simulink model "staticCalibrationDataGenerator"  (R2023b)
settings: Solver=VariableStepAuto  StartTime=0.0  StopTime=20  RelTol=1e-3
values from neighbouring files (symbols this model uses):
  acc_bias = [2*(rand-0.5)*acc_xy_bias_tolerance 2*(rand-0.5)*acc_xy_bias_tolerance 2*(rand-0.5)*acc_z_bias_tolerance]    [sim_cfg.m]
  acc_bias_over_temp = 2*(rand([1 3])-0.5)*acc_bias_over_temp_tolerance    [sim_cfg.m]
  acc_dynamic = 2*9.81    (= 19.62)    [sim_cfg.m]
  acc_freq = 100    [sim_cfg.m]
  acc_gain_over_temp = diag(2*(rand([1 3])-0.5)*acc_bias_over_temp_tolerance)    [sim_cfg.m]
  acc_noise = 0.008*9.81    (= 0.07848)    [sim_cfg.m]
  acc_non_orthogonality = acc_axis_alignement*acc_non_orthogonality    [sim_cfg.m]
  beac1_pos = [0.1 0 0]    [sim_cfg.m]
  beac2_pos = [-0.1 0 0]    [sim_cfg.m]
  cam1_k = X(39)    [calib2.m]    (also in der.m = C(8); sim_cfg.m = cam_res/(2*tan((cam_AoV+(rand-0.5)*cam_AoV_accur)/2)))
  cam1_orientation_q = angle2quat(cam1_orientation(1),cam1_orientation(2),cam1_orientation(3))    [sim_cfg.m]
  cam1_position = cam1_mounting_position+(rand([1 3])-0.5)*cam_mounting_accur_pos    [sim_cfg.m]
  cam2_k = X(47)    [calib2.m]    (also in der.m = C(16); sim_cfg.m = cam_res/(2*tan((cam_AoV+(rand-0.5)*cam_AoV_accur)/2)))
  cam2_orientation_q = angle2quat(cam2_orientation(1),cam2_orientation(2),cam2_orientation(3))    [sim_cfg.m]
  cam2_position = cam2_mounting_position+(rand([1 3])-0.5)*cam_mounting_accur_pos    [sim_cfg.m]
  cam_fps = 10    [sim_cfg.m]
  cam_noise = 1    [sim_cfg.m]
  cam_res = 480    [sim_cfg.m]
  f_sim = acc_freq    (= 100)    [sim_cfg.m]
  gps_freq = 20    [sim_cfg.m]
  gps_xy_noise = 0.1    [sim_cfg.m]
  gps_z_noise = 0.1    [sim_cfg.m]
  gravity = -9.812+(rand-0.5)*2*0.001    [sim_cfg.m]
  gyr_bias = 2*(rand([1 3])-0.5)*gyr_bias_tolerance    [sim_cfg.m]
  gyr_bias_over_temp = 2*(rand([1 3])-0.5)*gyr_bias_over_temp_tolerance    [sim_cfg.m]
  gyr_dynamic = 250*pi/180    (= 4.36332312999)    [sim_cfg.m]
  gyr_freq = 100    [sim_cfg.m]
  gyr_gain_over_temp = diag(2*(rand([1 3])-0.5)*gyr_bias_over_temp_tolerance)    [sim_cfg.m]
  gyr_noise = 0.1*pi/180    (= 0.00174532925199)    [sim_cfg.m]
  gyr_non_orthogonality = gyr_axis_alignement*gyr_non_orthogonality    [sim_cfg.m]
libraries: accelerometers x32, simulink x7, robotcorelib x1
settings Model: Creator=student  LastModifiedBy=robin
settings OptimizationCC: ReuseModelBlockBuffer=off

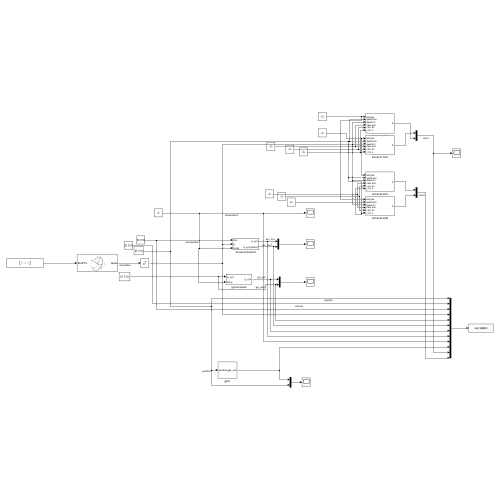
[thumbnail: Simulink's stored preview of the top-level diagram]
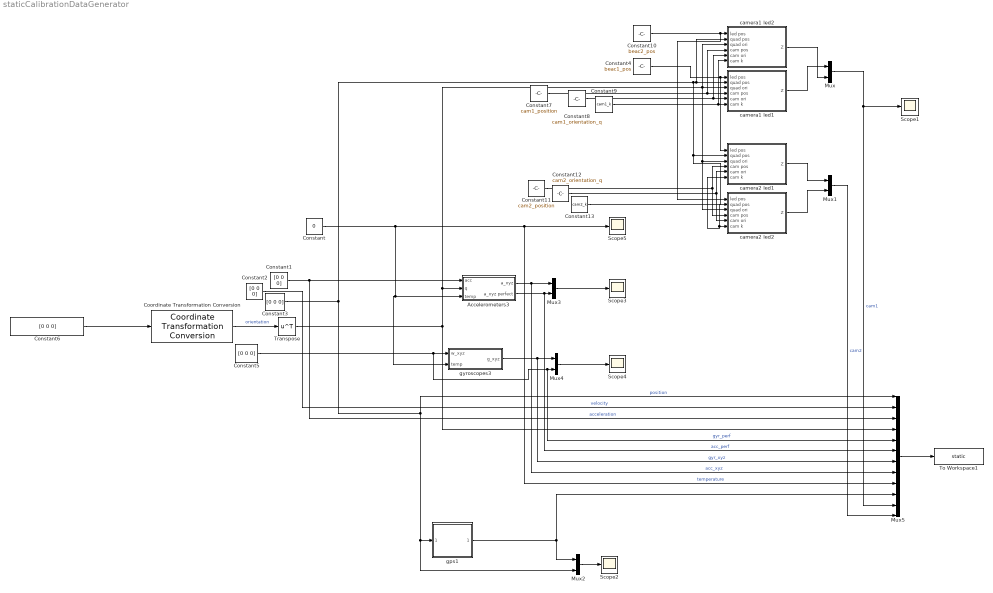
== system staticCalibrationDataGenerator ==
  Accelerometers3 : Subsystem
  Constant : Constant  Value=0
  Constant{1..3,5..6} (5 alike) : Constant  Value=[0 0 0]
  Constant10 : Constant  Value=beac2_pos
  Constant11 : Constant  Value=cam2_position
  Constant12 : Constant  Value=cam2_orientation_q
  Constant13 : Constant  Value=cam2_k
  Constant4 : Constant  Value=beac1_pos
  Constant7 : Constant  Value=cam1_position
  Constant8 : Constant  Value=cam1_orientation_q
  Constant9 : Constant  Value=cam1_k
  Coordinate Transformation Conversion : robotcorelib/Coordinate Transformation Conversion  InputRepresentation=Euler Angles  InputEulerSequence=ZYX  ShowTrVecInputPort=on  OutputRepresentation=Quaternion  OutputEulerSequence=ZYX  ShowTrVecOutputPort=on  SimulateUsing=Interpreted execution
      settings: LibrarySourceBlock=navlib/Utilities/Coordinate Transformation Conversion
  Mux{,1..4} (5 alike) : Mux  Inputs=2
  Mux5 : Mux  Inputs=12
  Scope{1..5} (5 alike) : Scope
  To Workspace1 : ToWorkspace  VariableName=static  SaveFormat=Structure With Time  SampleTime=1/f_sim
  Transpose : Math  Operator=transpose
  camera1 led1 : Subsystem  AncestorBlock=cam/camera led1
  camera1 led2 : Subsystem  AncestorBlock=cam/camera led1
  camera2 led1 : Subsystem  AncestorBlock=cam/camera led1
  camera2 led2 : Subsystem  AncestorBlock=cam/camera led1
  gps1 : Subsystem
  gyroscopes3 : Subsystem
  wires:
  Coordinate Transformation Conversion/1 -> Transpose/1  "orientation"
  Constant6/1 -> Coordinate Transformation Conversion/1
  Transpose/1 -> camera1 led1/3(quad ori), camera1 led2/3(quad ori), camera2 led2/3(quad ori), camera2 led1/3(quad ori), Accelerometers3/2(q), Mux5/4
  Accelerometers3/1(a_xyz) -> Mux5/8, Mux3/1  "acc_xyz"
  Constant5/1 -> gyroscopes3/1(w_xyz), Mux5/5, Mux4/2  "gyr_perf"
  Constant1/1 -> Accelerometers3/1(acc), Mux5/3  "acceleration"
  gyroscopes3/1(g_xyz) -> Mux5/7, Mux4/1  "gyr_xyz"
  Accelerometers3/2(a_xyz perfect) -> Mux5/6, Mux3/2  "acc_perf"
  Mux4/1 -> Scope4/1
  Constant/1 -> gyroscopes3/2(temp), Accelerometers3/3(temp), Scope5/1, Mux5/9  "temperature"
  Constant2/1 -> Mux5/2  "velocity"
  Mux3/1 -> Scope3/1
  Mux5/1 -> To Workspace1/1
  Constant3/1 -> camera1 led1/2(quad pos), camera1 led2/2(quad pos), camera2 led2/2(quad pos), camera2 led1/2(quad pos), Mux2/2, gps1/1(position), Mux5/1  "position"
  gps1/1(gps_out) -> Mux5/10, Mux2/1
  Mux2/1 -> Scope2/1
  Constant4/1 -> camera2 led1/1(led pos), camera1 led1/1(led pos)
  Constant7/1 -> camera1 led1/4(cam pos), camera1 led2/4(cam pos)
  Constant8/1 -> camera1 led1/5(cam ori), camera1 led2/5(cam ori)
  Constant9/1 -> camera1 led1/6(cam k), camera1 led2/6(cam k)
  Constant10/1 -> camera2 led2/1(led pos), camera1 led2/1(led pos)
  Constant13/1 -> camera2 led1/6(cam k), camera2 led2/6(cam k)
  Constant12/1 -> camera2 led2/5(cam ori), camera2 led1/5(cam ori)
  Constant11/1 -> camera2 led2/4(cam pos), camera2 led1/4(cam pos)
  camera2 led1/1(Z) -> Mux1/1
  camera2 led2/1(Z) -> Mux1/2
  Mux/1 -> Mux5/11, Scope1/1  "cam1"
  Mux1/1 -> Mux5/12  "cam2"
  camera1 led1/1(Z) -> Mux/1
  camera1 led2/1(Z) -> Mux/2

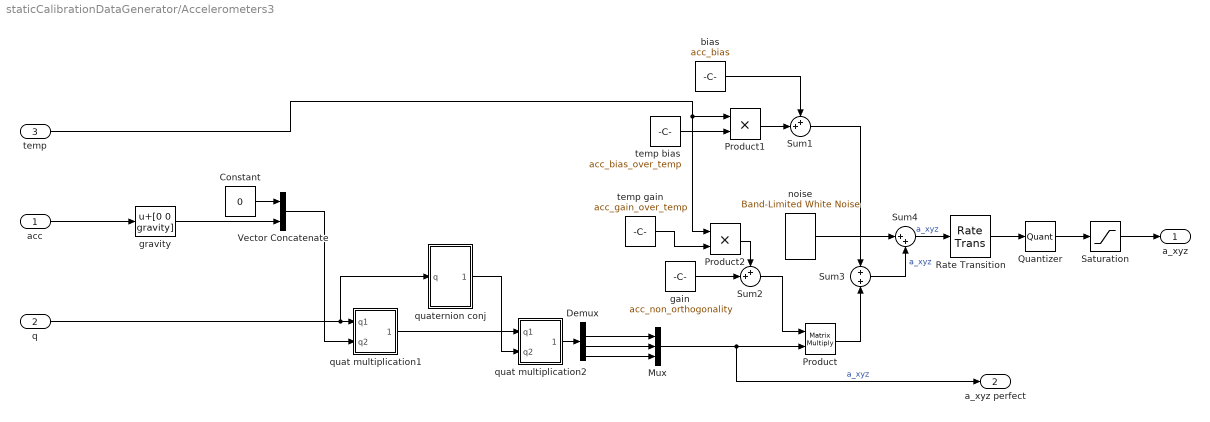
== system staticCalibrationDataGenerator/Accelerometers3 ==
  acc : Inport
  q : Inport  Port=2
  temp : Inport  Port=3
  Constant : Constant  Value=0
  Demux : Demux
  Mux : Mux  Inputs=3
  Product : Product  Multiplication=Matrix(*)
  Product1 : Product
  Product2 : Product
  Quantizer : Quantizer  QuantizationInterval=acc_res
  Rate Transition : RateTransition  OutPortSampleTime=1/acc_freq
  Saturation : Saturate  UpperLimit=acc_dynamic  LowerLimit=-acc_dynamic
  Sum1 : Sum  Inputs=++|
  Sum2 : Sum  Inputs=++|
  Sum3 : Sum
  Sum4 : Sum  Inputs=|++
  Vector Concatenate : Concatenate
  bias : Constant  Value=acc_bias
  gain : Constant  Value=acc_non_orthogonality
  gravity : Bias  Bias=[0 0 gravity]  SaturateOnIntegerOverflow=off
  noise : simulink/Sources/Band-Limited White Noise  Cov=[2*(2*pi*acc_noise/acc_freq)^2 2*(2*pi*acc_noise/acc_freq)^2 2*(2*pi*acc_noise/acc_freq)^2]  Ts=1/acc_freq  seed=[randi(1000) randi(1000) randi(1000)]  VectorParams1D=off
  quat multiplication1 : Subsystem
  quat multiplication2 : Subsystem
  quaternion conj : Subsystem
  temp bias : Constant  Value=acc_bias_over_temp
  temp gain : Constant  Value=acc_gain_over_temp
  a_xyz : Outport
  a_xyz perfect : Outport  Port=2
  wires:
  q/1 -> quat multiplication1/1(q1), quaternion conj/1(q)
  Sum4/1 -> Rate Transition/1  "a_xyz"
  Constant/1 -> Vector Concatenate/1
  Vector Concatenate/1 -> quat multiplication1/2(q2)
  gravity/1 -> Vector Concatenate/2
  quaternion conj/1(q conj) -> quat multiplication2/2(q2)
  quat multiplication1/1(q1*q2) -> quat multiplication2/1(q1)
  acc/1 -> gravity/1
  quat multiplication2/1(q1*q2) -> Demux/1
  Demux/2 -> Mux/1
  Demux/3 -> Mux/2
  Demux/4 -> Mux/3
  bias/1 -> Sum1/1
  Product1/1 -> Sum1/2
  temp bias/1 -> Product1/2
  temp/1 -> Product2/1, Product1/1
  temp gain/1 -> Product2/2
  gain/1 -> Sum2/2
  Sum2/1 -> Product/1
  Product2/1 -> Sum2/1
  Product/1 -> Sum3/2
  Sum1/1 -> Sum3/1
  Sum3/1 -> Sum4/2  "a_xyz"
  noise/1 -> Sum4/1
  Mux/1 -> a_xyz perfect/1, Product/2  "a_xyz"
  Saturation/1 -> a_xyz/1
  Rate Transition/1 -> Quantizer/1
  Quantizer/1 -> Saturation/1

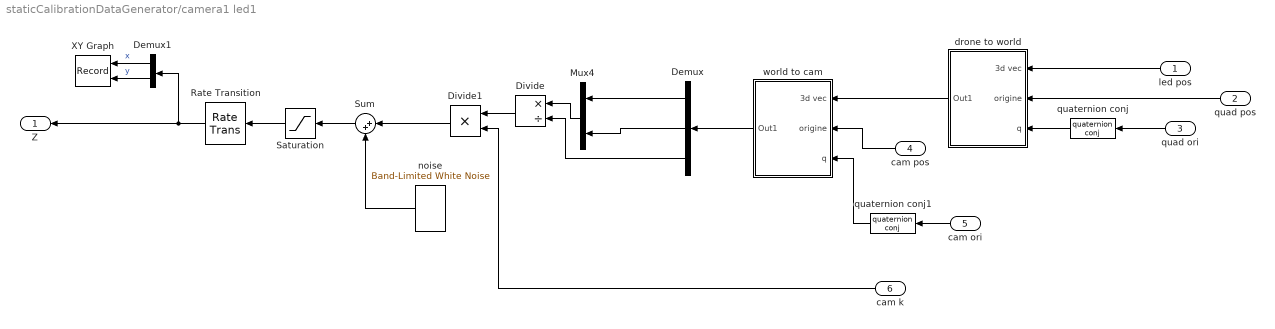
== system staticCalibrationDataGenerator/camera1 led1 ==
  led pos : Inport
  quad pos : Inport  Port=2
  quad ori : Inport  Port=3
  cam pos : Inport  Port=4
  cam ori : Inport  Port=5
  cam k : Inport  Port=6
  Demux : Demux  Outputs=3
  Demux1 : Demux  Outputs=2
  Divide : Product  Inputs=*/
  Divide1 : Product  Inputs=**
  Mux4 : Mux  Inputs=2
  Rate Transition : RateTransition  OutPortSampleTime=1/cam_fps
  Saturation : Saturate  UpperLimit=0.5*cam_res  LowerLimit=-0.5*cam_res  LinearizeAsGain=off
  Sum : Sum  Inputs=|++
  XY Graph : Record  FileSettingsInternal="{\"entries\":[{\"content\":{\"excelSettings\":{\"content\":{},\"type\":\"Streamout.ExcelSettings\"}},\"type\":\"Streamout.FileSettingStorage\",\"uuid\":\"\"}],\"packageUris\":[\"http:\\/\\/schema.mathworks.com\\/mf0\\/streamout_blocks\\/R2020a\"],\"version\":\"1.0\"}"  Layout=[1 1]  SignalsInternal="{\"entries\":[{\"content\":{\"signals\":[{\"content\":{\"blockPath\":[],\"dimensions\":[1,1],\"domain\":\"\",\"lineColor\":\"#ff6929\",\"port\":1,\"signalID\":145,\"signalName\":\"x\"},\"type\":\"RecordBlkView.Signal\",\"uuid\":\"\"},{\"content\":{\"blockPath\":[],\"dimensions\":[1,1],\"domain\":\"\",\"lineColor\":\"#b746ff\",\"port\":2,\"signalID\":148,\"signalName\":\"y\"},\"type\":\"RecordBlkView.Signal\",\"uuid\":\"\"}]},\"type\":\"RecordBlkView.InputSignals\",\"uuid\":\"\"}],\"packageUris\":[\"http:\\/\\/schema.mathworks.com\\/mf0\\/streamout_blocks\\/R2020a\"],\"version\":\"1.0\"}"  VisualizationBindings="{\"xyplotplugin\":{\"info\":[{\"series\":[],\"subplotID\":1}]}}"  CompatibilityTag=XY
  drone to world : Subsystem
  noise : simulink/Sources/Band-Limited White Noise  Cov="[(pi*cam_noise/cam_fps)^2  (pi*cam_noise/cam_fps)^2 ]"  Ts=1/cam_fps  seed=[randi(1020) randi(1030)]  VectorParams1D=off
  quaternion conj : accelerometers/accelerometer/quaternion conj  SystemSampleTime=-1  VariantActivationTime=update diagram  AllowFlexibleInterface=on  Latency=0  AutoFrameSizeCalculation=off
  quaternion conj1 : accelerometers/accelerometer/quaternion conj  SystemSampleTime=-1  VariantActivationTime=update diagram  AllowFlexibleInterface=on  Latency=0  AutoFrameSizeCalculation=off
  world to cam : Subsystem
  Z : Outport
  wires:
  quad ori/1 -> quaternion conj/1
  Demux/3 -> Divide/2
  cam ori/1 -> quaternion conj1/1
  world to cam/1(Out1) -> Demux/1
  Demux1/1 -> XY Graph/1  "x"
  Divide/1 -> Divide1/1
  Mux4/1 -> Divide/1
  Demux/2 -> Mux4/2
  Demux/1 -> Mux4/1
  Sum/1 -> Saturation/1
  noise/1 -> Sum/2
  Demux1/2 -> XY Graph/2  "y"
  Divide1/1 -> Sum/1
  cam pos/1 -> world to cam/2(origine)
  Saturation/1 -> Rate Transition/1
  quad pos/1 -> drone to world/2(origine)
  led pos/1 -> drone to world/1(3d vec)
  Rate Transition/1 -> Demux1/1, Z/1
  cam k/1 -> Divide1/2
  drone to world/1(Out1) -> world to cam/1(3d vec)
  quaternion conj/1 -> drone to world/3(q)
  quaternion conj1/1 -> world to cam/3(q)

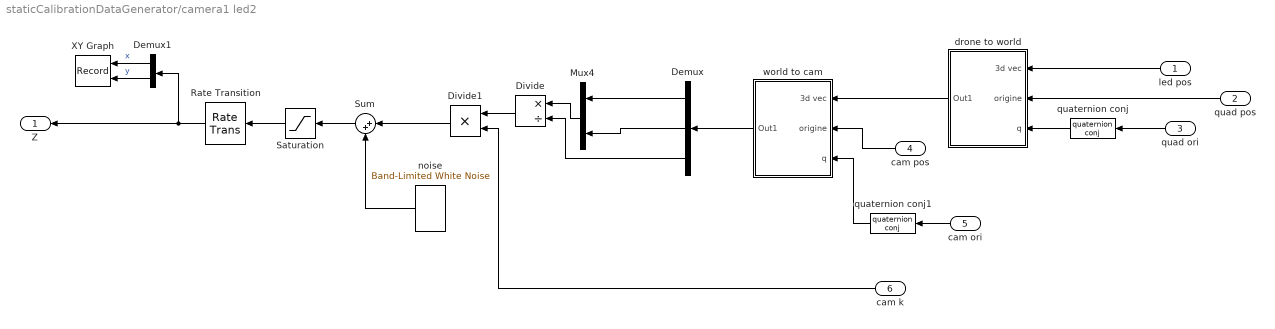
== system staticCalibrationDataGenerator/camera1 led2 ==
  led pos : Inport
  quad pos : Inport  Port=2
  quad ori : Inport  Port=3
  cam pos : Inport  Port=4
  cam ori : Inport  Port=5
  cam k : Inport  Port=6
  Demux : Demux  Outputs=3
  Demux1 : Demux  Outputs=2
  Divide : Product  Inputs=*/
  Divide1 : Product  Inputs=**
  Mux4 : Mux  Inputs=2
  Rate Transition : RateTransition  OutPortSampleTime=1/cam_fps
  Saturation : Saturate  UpperLimit=0.5*cam_res  LowerLimit=-0.5*cam_res  LinearizeAsGain=off
  Sum : Sum  Inputs=|++
  XY Graph : Record  FileSettingsInternal="{\"entries\":[{\"content\":{\"excelSettings\":{\"content\":{},\"type\":\"Streamout.ExcelSettings\"}},\"type\":\"Streamout.FileSettingStorage\",\"uuid\":\"\"}],\"packageUris\":[\"http:\\/\\/schema.mathworks.com\\/mf0\\/streamout_blocks\\/R2020a\"],\"version\":\"1.0\"}"  Layout=[1 1]  SignalsInternal="{\"entries\":[{\"content\":{\"signals\":[{\"content\":{\"blockPath\":[],\"dimensions\":[1,1],\"domain\":\"\",\"lineColor\":\"#ff13a6\",\"port\":1,\"signalID\":137,\"signalName\":\"x\"},\"type\":\"RecordBlkView.Signal\",\"uuid\":\"\"},{\"content\":{\"blockPath\":[],\"dimensions\":[1,1],\"domain\":\"\",\"lineColor\":\"#fe330a\",\"port\":2,\"signalID\":140,\"signalName\":\"y\"},\"type\":\"RecordBlkView.Signal\",\"uuid\":\"\"}]},\"type\":\"RecordBlkView.InputSignals\",\"uuid\":\"\"}],\"packageUris\":[\"http:\\/\\/schema.mathworks.com\\/mf0\\/streamout_blocks\\/R2020a\"],\"version\":\"1.0\"}"  VisualizationBindings="{\"xyplotplugin\":{\"info\":[{\"series\":[],\"subplotID\":1}]}}"  CompatibilityTag=XY
  drone to world : Subsystem
  noise : simulink/Sources/Band-Limited White Noise  Cov="[(pi*cam_noise/cam_fps)^2  (pi*cam_noise/cam_fps)^2 ]"  Ts=1/cam_fps  seed=[randi(1020) randi(1030)]  VectorParams1D=off
  quaternion conj : accelerometers/accelerometer/quaternion conj  SystemSampleTime=-1  VariantActivationTime=update diagram  AllowFlexibleInterface=on  Latency=0  AutoFrameSizeCalculation=off
  quaternion conj1 : accelerometers/accelerometer/quaternion conj  SystemSampleTime=-1  VariantActivationTime=update diagram  AllowFlexibleInterface=on  Latency=0  AutoFrameSizeCalculation=off
  world to cam : Subsystem
  Z : Outport
  wires:
  quad ori/1 -> quaternion conj/1
  Demux/3 -> Divide/2
  cam ori/1 -> quaternion conj1/1
  world to cam/1(Out1) -> Demux/1
  Demux1/1 -> XY Graph/1  "x"
  Divide/1 -> Divide1/1
  Mux4/1 -> Divide/1
  Demux/2 -> Mux4/2
  Demux/1 -> Mux4/1
  Sum/1 -> Saturation/1
  noise/1 -> Sum/2
  Demux1/2 -> XY Graph/2  "y"
  Divide1/1 -> Sum/1
  cam pos/1 -> world to cam/2(origine)
  Saturation/1 -> Rate Transition/1
  quad pos/1 -> drone to world/2(origine)
  led pos/1 -> drone to world/1(3d vec)
  Rate Transition/1 -> Demux1/1, Z/1
  cam k/1 -> Divide1/2
  drone to world/1(Out1) -> world to cam/1(3d vec)
  quaternion conj/1 -> drone to world/3(q)
  quaternion conj1/1 -> world to cam/3(q)

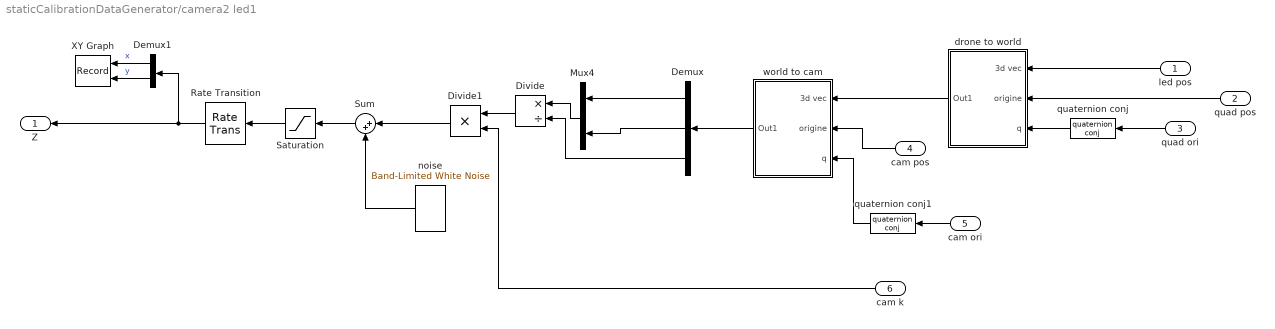
== system staticCalibrationDataGenerator/camera2 led1 ==
  led pos : Inport
  quad pos : Inport  Port=2
  quad ori : Inport  Port=3
  cam pos : Inport  Port=4
  cam ori : Inport  Port=5
  cam k : Inport  Port=6
  Demux : Demux  Outputs=3
  Demux1 : Demux  Outputs=2
  Divide : Product  Inputs=*/
  Divide1 : Product  Inputs=**
  Mux4 : Mux  Inputs=2
  Rate Transition : RateTransition  OutPortSampleTime=1/cam_fps
  Saturation : Saturate  UpperLimit=0.5*cam_res  LowerLimit=-0.5*cam_res  LinearizeAsGain=off
  Sum : Sum  Inputs=|++
  XY Graph : Record  FileSettingsInternal="{\"entries\":[{\"content\":{\"excelSettings\":{\"content\":{},\"type\":\"Streamout.ExcelSettings\"}},\"type\":\"Streamout.FileSettingStorage\",\"uuid\":\"\"}],\"packageUris\":[\"http:\\/\\/schema.mathworks.com\\/mf0\\/streamout_blocks\\/R2020a\"],\"version\":\"1.0\"}"  Layout=[1 1]  SignalsInternal="{\"entries\":[{\"content\":{\"signals\":[{\"content\":{\"blockPath\":[],\"dimensions\":[1,1],\"domain\":\"\",\"lineColor\":\"#0072bd\",\"port\":1,\"signalID\":129,\"signalName\":\"x\"},\"type\":\"RecordBlkView.Signal\",\"uuid\":\"\"},{\"content\":{\"blockPath\":[],\"dimensions\":[1,1],\"domain\":\"\",\"lineColor\":\"#d95319\",\"port\":2,\"signalID\":132,\"signalName\":\"y\"},\"type\":\"RecordBlkView.Signal\",\"uuid\":\"\"}]},\"type\":\"RecordBlkView.InputSignals\",\"uuid\":\"\"}],\"packageUris\":[\"http:\\/\\/schema.mathworks.com\\/mf0\\/streamout_blocks\\/R2020a\"],\"version\":\"1.0\"}"  VisualizationBindings="{\"xyplotplugin\":{\"info\":[{\"series\":[],\"subplotID\":1}]}}"  CompatibilityTag=XY
  drone to world : Subsystem
  noise : simulink/Sources/Band-Limited White Noise  Cov="[(pi*cam_noise/cam_fps)^2  (pi*cam_noise/cam_fps)^2 ]"  Ts=1/cam_fps  seed=[randi(1020) randi(1030)]  VectorParams1D=off
  quaternion conj : accelerometers/accelerometer/quaternion conj  SystemSampleTime=-1  VariantActivationTime=update diagram  AllowFlexibleInterface=on  Latency=0  AutoFrameSizeCalculation=off
  quaternion conj1 : accelerometers/accelerometer/quaternion conj  SystemSampleTime=-1  VariantActivationTime=update diagram  AllowFlexibleInterface=on  Latency=0  AutoFrameSizeCalculation=off
  world to cam : Subsystem
  Z : Outport
  wires:
  quad ori/1 -> quaternion conj/1
  Demux/3 -> Divide/2
  cam ori/1 -> quaternion conj1/1
  world to cam/1(Out1) -> Demux/1
  Demux1/1 -> XY Graph/1  "x"
  Divide/1 -> Divide1/1
  Mux4/1 -> Divide/1
  Demux/2 -> Mux4/2
  Demux/1 -> Mux4/1
  Sum/1 -> Saturation/1
  noise/1 -> Sum/2
  Demux1/2 -> XY Graph/2  "y"
  Divide1/1 -> Sum/1
  cam pos/1 -> world to cam/2(origine)
  Saturation/1 -> Rate Transition/1
  quad pos/1 -> drone to world/2(origine)
  led pos/1 -> drone to world/1(3d vec)
  Rate Transition/1 -> Demux1/1, Z/1
  cam k/1 -> Divide1/2
  drone to world/1(Out1) -> world to cam/1(3d vec)
  quaternion conj/1 -> drone to world/3(q)
  quaternion conj1/1 -> world to cam/3(q)

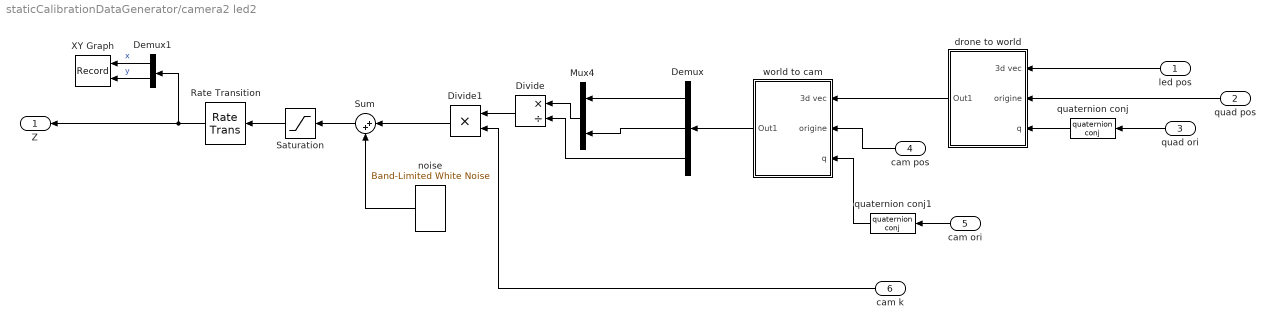
== system staticCalibrationDataGenerator/camera2 led2 ==
  led pos : Inport
  quad pos : Inport  Port=2
  quad ori : Inport  Port=3
  cam pos : Inport  Port=4
  cam ori : Inport  Port=5
  cam k : Inport  Port=6
  Demux : Demux  Outputs=3
  Demux1 : Demux  Outputs=2
  Divide : Product  Inputs=*/
  Divide1 : Product  Inputs=**
  Mux4 : Mux  Inputs=2
  Rate Transition : RateTransition  OutPortSampleTime=1/cam_fps
  Saturation : Saturate  UpperLimit=0.5*cam_res  LowerLimit=-0.5*cam_res  LinearizeAsGain=off
  Sum : Sum  Inputs=|++
  XY Graph : Record  FileSettingsInternal="{\"entries\":[{\"content\":{\"excelSettings\":{\"content\":{},\"type\":\"Streamout.ExcelSettings\"}},\"type\":\"Streamout.FileSettingStorage\",\"uuid\":\"\"}],\"packageUris\":[\"http:\\/\\/schema.mathworks.com\\/mf0\\/streamout_blocks\\/R2020a\"],\"version\":\"1.0\"}"  Layout=[1 1]  SignalsInternal="{\"entries\":[{\"content\":{\"signals\":[{\"content\":{\"blockPath\":[],\"dimensions\":[1,1],\"domain\":\"\",\"lineColor\":\"#7e2f8e\",\"port\":1,\"signalID\":153,\"signalName\":\"x\"},\"type\":\"RecordBlkView.Signal\",\"uuid\":\"\"},{\"content\":{\"blockPath\":[],\"dimensions\":[1,1],\"domain\":\"\",\"lineColor\":\"#77ac30\",\"port\":2,\"signalID\":156,\"signalName\":\"y\"},\"type\":\"RecordBlkView.Signal\",\"uuid\":\"\"}]},\"type\":\"RecordBlkView.InputSignals\",\"uuid\":\"\"}],\"packageUris\":[\"http:\\/\\/schema.mathworks.com\\/mf0\\/streamout_blocks\\/R2020a\"],\"version\":\"1.0\"}"  VisualizationBindings="{\"xyplotplugin\":{\"info\":[{\"series\":[],\"subplotID\":1}]}}"  CompatibilityTag=XY
  drone to world : Subsystem
  noise : simulink/Sources/Band-Limited White Noise  Cov="[(pi*cam_noise/cam_fps)^2  (pi*cam_noise/cam_fps)^2 ]"  Ts=1/cam_fps  seed=[randi(1020) randi(1030)]  VectorParams1D=off
  quaternion conj : accelerometers/accelerometer/quaternion conj  SystemSampleTime=-1  VariantActivationTime=update diagram  AllowFlexibleInterface=on  Latency=0  AutoFrameSizeCalculation=off
  quaternion conj1 : accelerometers/accelerometer/quaternion conj  SystemSampleTime=-1  VariantActivationTime=update diagram  AllowFlexibleInterface=on  Latency=0  AutoFrameSizeCalculation=off
  world to cam : Subsystem
  Z : Outport
  wires:
  quad ori/1 -> quaternion conj/1
  Demux/3 -> Divide/2
  cam ori/1 -> quaternion conj1/1
  world to cam/1(Out1) -> Demux/1
  Demux1/1 -> XY Graph/1  "x"
  Divide/1 -> Divide1/1
  Mux4/1 -> Divide/1
  Demux/2 -> Mux4/2
  Demux/1 -> Mux4/1
  Sum/1 -> Saturation/1
  noise/1 -> Sum/2
  Demux1/2 -> XY Graph/2  "y"
  Divide1/1 -> Sum/1
  cam pos/1 -> world to cam/2(origine)
  Saturation/1 -> Rate Transition/1
  quad pos/1 -> drone to world/2(origine)
  led pos/1 -> drone to world/1(3d vec)
  Rate Transition/1 -> Demux1/1, Z/1
  cam k/1 -> Divide1/2
  drone to world/1(Out1) -> world to cam/1(3d vec)
  quaternion conj/1 -> drone to world/3(q)
  quaternion conj1/1 -> world to cam/3(q)

== system staticCalibrationDataGenerator/gps1 ==
  position : Inport
  Band-Limited White Noise1 : simulink/Sources/Band-Limited White Noise  Cov=[2*(2*pi*gps_xy_noise/gps_freq)^2 2*(2*pi*gps_xy_noise/gps_freq)^2 2*(2*pi*gps_z_noise/gps_freq)^2]  Ts=1/gps_freq  seed=[randi(10000) randi(10000) randi(10000)]  VectorParams1D=off
  Quantizer : Quantizer  QuantizationInterval=gps_res
  Rate Transition : RateTransition  OutPortSampleTime=1/gps_freq
  Sum3 : Sum  Inputs=++|
  gps_out : Outport
  wires:
  Rate Transition/1 -> Quantizer/1
  Quantizer/1 -> gps_out/1
  Band-Limited White Noise1/1 -> Sum3/1
  Sum3/1 -> Rate Transition/1
  position/1 -> Sum3/2

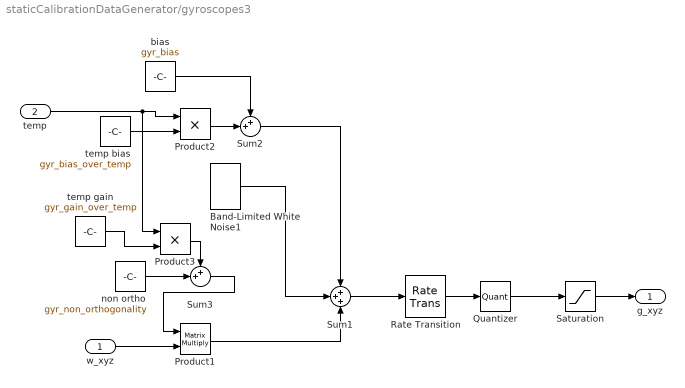
== system staticCalibrationDataGenerator/gyroscopes3 ==
  w_xyz : Inport
  temp : Inport  Port=2
  Band-Limited White Noise1 : simulink/Sources/Band-Limited White Noise  Cov=[2*(2*pi*gyr_noise/gyr_freq)^2 2*(2*pi*gyr_noise/gyr_freq)^2 2*(2*pi*gyr_noise/gyr_freq)^2]  Ts=1/gyr_freq  seed=[randi(1000) randi(1000) randi(1000)]  VectorParams1D=off
  Product1 : Product  Multiplication=Matrix(*)
  Product2 : Product
  Product3 : Product
  Quantizer : Quantizer  QuantizationInterval=gyr_res
  Rate Transition : RateTransition  OutPortSampleTime=1/gyr_freq
  Saturation : Saturate  UpperLimit=gyr_dynamic  LowerLimit=-gyr_dynamic
  Sum1 : Sum  Inputs=+++
  Sum2 : Sum  Inputs=++|
  Sum3 : Sum  Inputs=++|
  bias : Constant  Value=gyr_bias
  non ortho : Constant  Value=gyr_non_orthogonality
  temp bias : Constant  Value=gyr_bias_over_temp
  temp gain : Constant  Value=gyr_gain_over_temp
  g_xyz : Outport
  wires:
  non ortho/1 -> Sum3/2
  Product3/1 -> Sum3/1
  temp/1 -> Product3/1, Product2/1
  Product2/1 -> Sum2/2
  temp gain/1 -> Product3/2
  temp bias/1 -> Product2/2
  Sum3/1 -> Product1/1
  bias/1 -> Sum2/1
  Band-Limited White Noise1/1 -> Sum1/2
  Sum2/1 -> Sum1/1
  w_xyz/1 -> Product1/2
  Product1/1 -> Sum1/3
  Saturation/1 -> g_xyz/1
  Rate Transition/1 -> Quantizer/1
  Sum1/1 -> Rate Transition/1
  Quantizer/1 -> Saturation/1

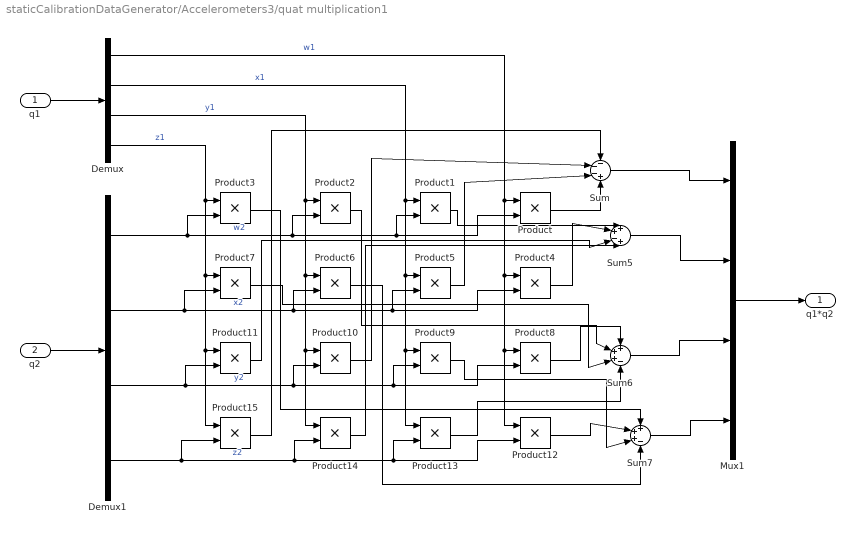
== system staticCalibrationDataGenerator/Accelerometers3/quat multiplication1 ==
  q1 : Inport
  q2 : Inport  Port=2
  Demux : Demux
  Demux1 : Demux
  Mux1 : Mux
  Product{,1..15} (16 alike) : Product
  Sum : Sum  Inputs=---+
  Sum5 : Sum  Inputs=++-+
  Sum6 : Sum  Inputs=+++-
  Sum7 : Sum  Inputs=+++-
  q1*q2 : Outport
  wires:
  Sum5/1 -> Mux1/2
  Product/1 -> Sum/4
  Product9/1 -> Sum7/3
  Demux/1 -> Product12/1, Product8/1, Product4/1, Product/1  "w1"
  Demux1/3 -> Product8/2, Product9/2, Product10/2, Product11/2  "y2"
  Demux/2 -> Product13/1, Product9/1, Product5/1, Product1/1  "x1"
  Product6/1 -> Sum7/4
  Product4/1 -> Sum5/2
  Demux1/1 -> Product/2, Product1/2, Product2/2, Product3/2  "w2"
  Sum/1 -> Mux1/1
  Product3/1 -> Sum7/1
  Product15/1 -> Sum/1
  Product1/1 -> Sum5/1
  Product2/1 -> Sum6/2
  Demux/4 -> Product15/1, Product11/1, Product7/1, Product3/1  "z1"
  Sum6/1 -> Mux1/3
  Demux1/2 -> Product4/2, Product5/2, Product6/2, Product7/2  "x2"
  Demux1/4 -> Product12/2, Product13/2, Product14/2, Product15/2  "z2"
  Product14/1 -> Sum5/4
  Mux1/1 -> q1*q2/1
  Sum7/1 -> Mux1/4
  Demux/3 -> Product14/1, Product10/1, Product6/1, Product2/1  "y1"
  Product13/1 -> Sum6/4
  Product8/1 -> Sum6/1
  q2/1 -> Demux1/1
  q1/1 -> Demux/1
  Product11/1 -> Sum5/3
  Product7/1 -> Sum6/3
  Product10/1 -> Sum/2
  Product5/1 -> Sum/3
  Product12/1 -> Sum7/2

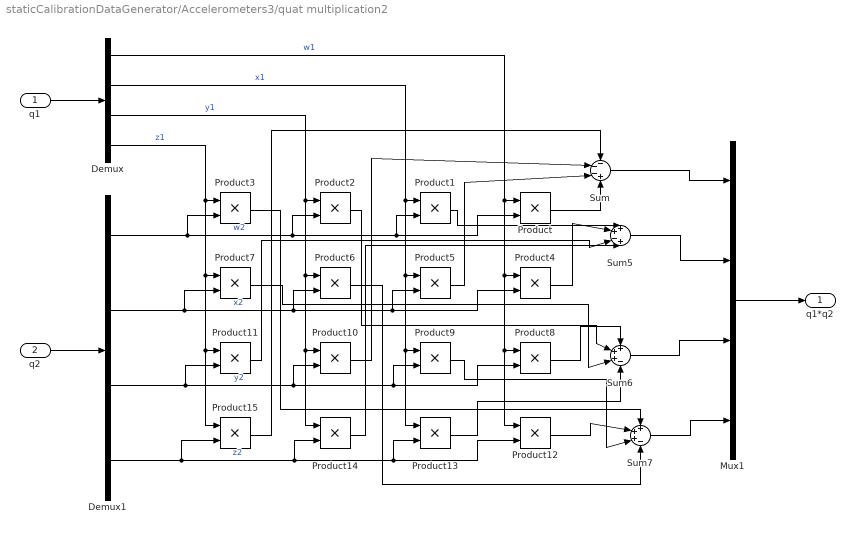
== system staticCalibrationDataGenerator/Accelerometers3/quat multiplication2 ==
  q1 : Inport
  q2 : Inport  Port=2
  Demux : Demux
  Demux1 : Demux
  Mux1 : Mux
  Product{,1..15} (16 alike) : Product
  Sum : Sum  Inputs=---+
  Sum5 : Sum  Inputs=++-+
  Sum6 : Sum  Inputs=+++-
  Sum7 : Sum  Inputs=+++-
  q1*q2 : Outport
  wires:
  Sum5/1 -> Mux1/2
  Product/1 -> Sum/4
  Product9/1 -> Sum7/3
  Demux/1 -> Product12/1, Product8/1, Product4/1, Product/1  "w1"
  Demux1/3 -> Product8/2, Product9/2, Product10/2, Product11/2  "y2"
  Demux/2 -> Product13/1, Product9/1, Product5/1, Product1/1  "x1"
  Product6/1 -> Sum7/4
  Product4/1 -> Sum5/2
  Demux1/1 -> Product/2, Product1/2, Product2/2, Product3/2  "w2"
  Sum/1 -> Mux1/1
  Product3/1 -> Sum7/1
  Product15/1 -> Sum/1
  Product1/1 -> Sum5/1
  Product2/1 -> Sum6/2
  Demux/4 -> Product15/1, Product11/1, Product7/1, Product3/1  "z1"
  Sum6/1 -> Mux1/3
  Demux1/2 -> Product4/2, Product5/2, Product6/2, Product7/2  "x2"
  Demux1/4 -> Product12/2, Product13/2, Product14/2, Product15/2  "z2"
  Product14/1 -> Sum5/4
  Mux1/1 -> q1*q2/1
  Sum7/1 -> Mux1/4
  Demux/3 -> Product14/1, Product10/1, Product6/1, Product2/1  "y1"
  Product13/1 -> Sum6/4
  Product8/1 -> Sum6/1
  q2/1 -> Demux1/1
  q1/1 -> Demux/1
  Product11/1 -> Sum5/3
  Product7/1 -> Sum6/3
  Product10/1 -> Sum/2
  Product5/1 -> Sum/3
  Product12/1 -> Sum7/2

== system staticCalibrationDataGenerator/Accelerometers3/quaternion conj ==
  q : Inport
  Demux : Demux
  Gain : Gain  Gain=-1
  Gain2 : Gain  Gain=-1
  Gain3 : Gain  Gain=-1
  Mux : Mux
  q conj : Outport
  wires:
  Gain2/1 -> Mux/3
  Demux/3 -> Gain2/1  "y1"
  Demux/1 -> Mux/1  "w1"
  Gain3/1 -> Mux/4
  Demux/4 -> Gain3/1  "z1"
  q/1 -> Demux/1
  Mux/1 -> q conj/1
  Demux/2 -> Gain/1  "x1"
  Gain/1 -> Mux/2

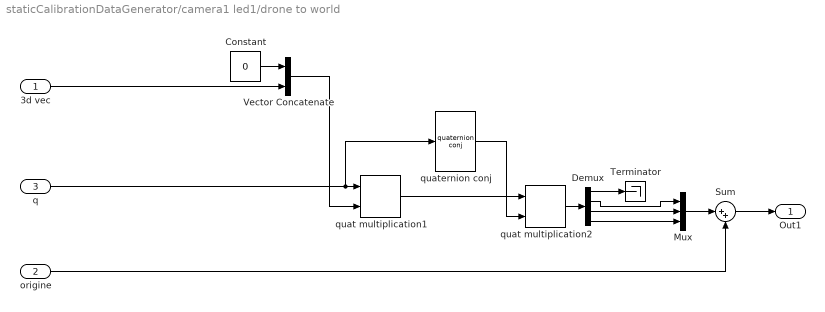
== system staticCalibrationDataGenerator/camera1 led1/drone to world ==
  3d vec : Inport
  origine : Inport  Port=2
  q : Inport  Port=3
  Constant : Constant  Value=0
  Demux : Demux
  Mux : Mux  Inputs=3
  Sum : Sum  Inputs=|++
  Terminator : Terminator
  Vector Concatenate : Concatenate
  quat multiplication1 : accelerometers/accelerometer/quat multiplication1  SystemSampleTime=-1  VariantActivationTime=update diagram  AllowFlexibleInterface=on  Latency=0  AutoFrameSizeCalculation=off
  quat multiplication2 : accelerometers/accelerometer/quat multiplication2  SystemSampleTime=-1  VariantActivationTime=update diagram  AllowFlexibleInterface=on  Latency=0  AutoFrameSizeCalculation=off
  quaternion conj : accelerometers/accelerometer/quaternion conj  SystemSampleTime=-1  VariantActivationTime=update diagram  AllowFlexibleInterface=on  Latency=0  AutoFrameSizeCalculation=off
  Out1 : Outport
  wires:
  Demux/1 -> Terminator/1
  Vector Concatenate/1 -> quat multiplication1/2
  quaternion conj/1 -> quat multiplication2/2
  quat multiplication2/1 -> Demux/1
  Constant/1 -> Vector Concatenate/1
  q/1 -> quaternion conj/1, quat multiplication1/1
  quat multiplication1/1 -> quat multiplication2/1
  Demux/3 -> Mux/2
  Demux/4 -> Mux/3
  Demux/2 -> Mux/1
  3d vec/1 -> Vector Concatenate/2
  Mux/1 -> Sum/1
  Sum/1 -> Out1/1
  origine/1 -> Sum/2

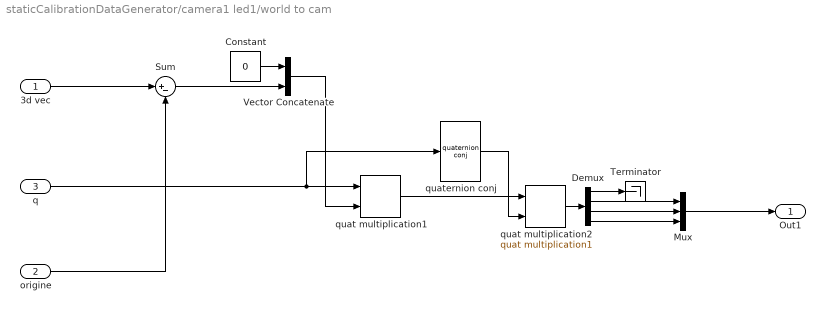
== system staticCalibrationDataGenerator/camera1 led1/world to cam ==
  3d vec : Inport
  origine : Inport  Port=2
  q : Inport  Port=3
  Constant : Constant  Value=0
  Demux : Demux
  Mux : Mux  Inputs=3
  Sum : Sum  Inputs=|+-
  Terminator : Terminator
  Vector Concatenate : Concatenate
  quat multiplication1 : accelerometers/accelerometer/quat multiplication1  SystemSampleTime=-1  VariantActivationTime=update diagram  AllowFlexibleInterface=on  Latency=0  AutoFrameSizeCalculation=off
  quat multiplication2 : accelerometers/accelerometer/quat multiplication1  SystemSampleTime=-1  VariantActivationTime=update diagram  AllowFlexibleInterface=on  Latency=0  AutoFrameSizeCalculation=off
  quaternion conj : accelerometers/accelerometer/quaternion conj  SystemSampleTime=-1  VariantActivationTime=update diagram  AllowFlexibleInterface=on  Latency=0  AutoFrameSizeCalculation=off
  Out1 : Outport
  wires:
  quat multiplication2/1 -> Demux/1
  Constant/1 -> Vector Concatenate/1
  Mux/1 -> Out1/1
  origine/1 -> Sum/2
  3d vec/1 -> Sum/1
  Sum/1 -> Vector Concatenate/2
  Vector Concatenate/1 -> quat multiplication1/2
  q/1 -> quaternion conj/1, quat multiplication1/1
  quat multiplication1/1 -> quat multiplication2/1
  quaternion conj/1 -> quat multiplication2/2
  Demux/2 -> Mux/1
  Demux/3 -> Mux/2
  Demux/4 -> Mux/3
  Demux/1 -> Terminator/1

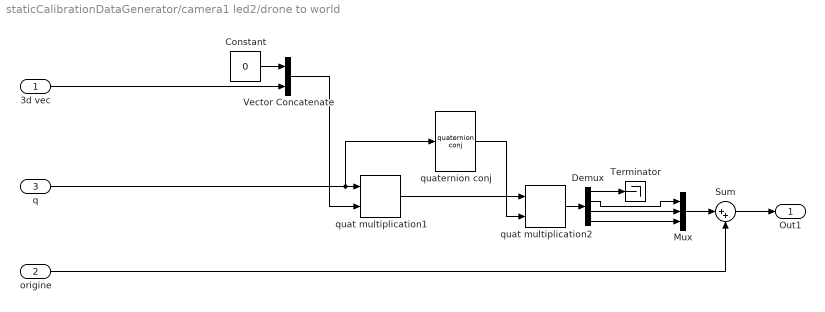
== system staticCalibrationDataGenerator/camera1 led2/drone to world ==
  3d vec : Inport
  origine : Inport  Port=2
  q : Inport  Port=3
  Constant : Constant  Value=0
  Demux : Demux
  Mux : Mux  Inputs=3
  Sum : Sum  Inputs=|++
  Terminator : Terminator
  Vector Concatenate : Concatenate
  quat multiplication1 : accelerometers/accelerometer/quat multiplication1  SystemSampleTime=-1  VariantActivationTime=update diagram  AllowFlexibleInterface=on  Latency=0  AutoFrameSizeCalculation=off
  quat multiplication2 : accelerometers/accelerometer/quat multiplication2  SystemSampleTime=-1  VariantActivationTime=update diagram  AllowFlexibleInterface=on  Latency=0  AutoFrameSizeCalculation=off
  quaternion conj : accelerometers/accelerometer/quaternion conj  SystemSampleTime=-1  VariantActivationTime=update diagram  AllowFlexibleInterface=on  Latency=0  AutoFrameSizeCalculation=off
  Out1 : Outport
  wires:
  Demux/1 -> Terminator/1
  Vector Concatenate/1 -> quat multiplication1/2
  quaternion conj/1 -> quat multiplication2/2
  quat multiplication2/1 -> Demux/1
  Constant/1 -> Vector Concatenate/1
  q/1 -> quaternion conj/1, quat multiplication1/1
  quat multiplication1/1 -> quat multiplication2/1
  Demux/3 -> Mux/2
  Demux/4 -> Mux/3
  Demux/2 -> Mux/1
  3d vec/1 -> Vector Concatenate/2
  Mux/1 -> Sum/1
  Sum/1 -> Out1/1
  origine/1 -> Sum/2

== system staticCalibrationDataGenerator/camera1 led2/world to cam ==
  3d vec : Inport
  origine : Inport  Port=2
  q : Inport  Port=3
  Constant : Constant  Value=0
  Demux : Demux
  Mux : Mux  Inputs=3
  Sum : Sum  Inputs=|+-
  Terminator : Terminator
  Vector Concatenate : Concatenate
  quat multiplication1 : accelerometers/accelerometer/quat multiplication1  SystemSampleTime=-1  VariantActivationTime=update diagram  AllowFlexibleInterface=on  Latency=0  AutoFrameSizeCalculation=off
  quat multiplication2 : accelerometers/accelerometer/quat multiplication1  SystemSampleTime=-1  VariantActivationTime=update diagram  AllowFlexibleInterface=on  Latency=0  AutoFrameSizeCalculation=off
  quaternion conj : accelerometers/accelerometer/quaternion conj  SystemSampleTime=-1  VariantActivationTime=update diagram  AllowFlexibleInterface=on  Latency=0  AutoFrameSizeCalculation=off
  Out1 : Outport
  wires:
  quat multiplication2/1 -> Demux/1
  Constant/1 -> Vector Concatenate/1
  Mux/1 -> Out1/1
  origine/1 -> Sum/2
  3d vec/1 -> Sum/1
  Sum/1 -> Vector Concatenate/2
  Vector Concatenate/1 -> quat multiplication1/2
  q/1 -> quaternion conj/1, quat multiplication1/1
  quat multiplication1/1 -> quat multiplication2/1
  quaternion conj/1 -> quat multiplication2/2
  Demux/2 -> Mux/1
  Demux/3 -> Mux/2
  Demux/4 -> Mux/3
  Demux/1 -> Terminator/1

== system staticCalibrationDataGenerator/camera2 led1/drone to world ==
  3d vec : Inport
  origine : Inport  Port=2
  q : Inport  Port=3
  Constant : Constant  Value=0
  Demux : Demux
  Mux : Mux  Inputs=3
  Sum : Sum  Inputs=|++
  Terminator : Terminator
  Vector Concatenate : Concatenate
  quat multiplication1 : accelerometers/accelerometer/quat multiplication1  SystemSampleTime=-1  VariantActivationTime=update diagram  AllowFlexibleInterface=on  Latency=0  AutoFrameSizeCalculation=off
  quat multiplication2 : accelerometers/accelerometer/quat multiplication2  SystemSampleTime=-1  VariantActivationTime=update diagram  AllowFlexibleInterface=on  Latency=0  AutoFrameSizeCalculation=off
  quaternion conj : accelerometers/accelerometer/quaternion conj  SystemSampleTime=-1  VariantActivationTime=update diagram  AllowFlexibleInterface=on  Latency=0  AutoFrameSizeCalculation=off
  Out1 : Outport
  wires:
  Demux/1 -> Terminator/1
  Vector Concatenate/1 -> quat multiplication1/2
  quaternion conj/1 -> quat multiplication2/2
  quat multiplication2/1 -> Demux/1
  Constant/1 -> Vector Concatenate/1
  q/1 -> quaternion conj/1, quat multiplication1/1
  quat multiplication1/1 -> quat multiplication2/1
  Demux/3 -> Mux/2
  Demux/4 -> Mux/3
  Demux/2 -> Mux/1
  3d vec/1 -> Vector Concatenate/2
  Mux/1 -> Sum/1
  Sum/1 -> Out1/1
  origine/1 -> Sum/2

== system staticCalibrationDataGenerator/camera2 led1/world to cam ==
  3d vec : Inport
  origine : Inport  Port=2
  q : Inport  Port=3
  Constant : Constant  Value=0
  Demux : Demux
  Mux : Mux  Inputs=3
  Sum : Sum  Inputs=|+-
  Terminator : Terminator
  Vector Concatenate : Concatenate
  quat multiplication1 : accelerometers/accelerometer/quat multiplication1  SystemSampleTime=-1  VariantActivationTime=update diagram  AllowFlexibleInterface=on  Latency=0  AutoFrameSizeCalculation=off
  quat multiplication2 : accelerometers/accelerometer/quat multiplication1  SystemSampleTime=-1  VariantActivationTime=update diagram  AllowFlexibleInterface=on  Latency=0  AutoFrameSizeCalculation=off
  quaternion conj : accelerometers/accelerometer/quaternion conj  SystemSampleTime=-1  VariantActivationTime=update diagram  AllowFlexibleInterface=on  Latency=0  AutoFrameSizeCalculation=off
  Out1 : Outport
  wires:
  quat multiplication2/1 -> Demux/1
  Constant/1 -> Vector Concatenate/1
  Mux/1 -> Out1/1
  origine/1 -> Sum/2
  3d vec/1 -> Sum/1
  Sum/1 -> Vector Concatenate/2
  Vector Concatenate/1 -> quat multiplication1/2
  q/1 -> quaternion conj/1, quat multiplication1/1
  quat multiplication1/1 -> quat multiplication2/1
  quaternion conj/1 -> quat multiplication2/2
  Demux/2 -> Mux/1
  Demux/3 -> Mux/2
  Demux/4 -> Mux/3
  Demux/1 -> Terminator/1

== system staticCalibrationDataGenerator/camera2 led2/drone to world ==
  3d vec : Inport
  origine : Inport  Port=2
  q : Inport  Port=3
  Constant : Constant  Value=0
  Demux : Demux
  Mux : Mux  Inputs=3
  Sum : Sum  Inputs=|++
  Terminator : Terminator
  Vector Concatenate : Concatenate
  quat multiplication1 : accelerometers/accelerometer/quat multiplication1  SystemSampleTime=-1  VariantActivationTime=update diagram  AllowFlexibleInterface=on  Latency=0  AutoFrameSizeCalculation=off
  quat multiplication2 : accelerometers/accelerometer/quat multiplication2  SystemSampleTime=-1  VariantActivationTime=update diagram  AllowFlexibleInterface=on  Latency=0  AutoFrameSizeCalculation=off
  quaternion conj : accelerometers/accelerometer/quaternion conj  SystemSampleTime=-1  VariantActivationTime=update diagram  AllowFlexibleInterface=on  Latency=0  AutoFrameSizeCalculation=off
  Out1 : Outport
  wires:
  Demux/1 -> Terminator/1
  Vector Concatenate/1 -> quat multiplication1/2
  quaternion conj/1 -> quat multiplication2/2
  quat multiplication2/1 -> Demux/1
  Constant/1 -> Vector Concatenate/1
  q/1 -> quaternion conj/1, quat multiplication1/1
  quat multiplication1/1 -> quat multiplication2/1
  Demux/3 -> Mux/2
  Demux/4 -> Mux/3
  Demux/2 -> Mux/1
  3d vec/1 -> Vector Concatenate/2
  Mux/1 -> Sum/1
  Sum/1 -> Out1/1
  origine/1 -> Sum/2

== system staticCalibrationDataGenerator/camera2 led2/world to cam ==
  3d vec : Inport
  origine : Inport  Port=2
  q : Inport  Port=3
  Constant : Constant  Value=0
  Demux : Demux
  Mux : Mux  Inputs=3
  Sum : Sum  Inputs=|+-
  Terminator : Terminator
  Vector Concatenate : Concatenate
  quat multiplication1 : accelerometers/accelerometer/quat multiplication1  SystemSampleTime=-1  VariantActivationTime=update diagram  AllowFlexibleInterface=on  Latency=0  AutoFrameSizeCalculation=off
  quat multiplication2 : accelerometers/accelerometer/quat multiplication1  SystemSampleTime=-1  VariantActivationTime=update diagram  AllowFlexibleInterface=on  Latency=0  AutoFrameSizeCalculation=off
  quaternion conj : accelerometers/accelerometer/quaternion conj  SystemSampleTime=-1  VariantActivationTime=update diagram  AllowFlexibleInterface=on  Latency=0  AutoFrameSizeCalculation=off
  Out1 : Outport
  wires:
  quat multiplication2/1 -> Demux/1
  Constant/1 -> Vector Concatenate/1
  Mux/1 -> Out1/1
  origine/1 -> Sum/2
  3d vec/1 -> Sum/1
  Sum/1 -> Vector Concatenate/2
  Vector Concatenate/1 -> quat multiplication1/2
  q/1 -> quaternion conj/1, quat multiplication1/1
  quat multiplication1/1 -> quat multiplication2/1
  quaternion conj/1 -> quat multiplication2/2
  Demux/2 -> Mux/1
  Demux/3 -> Mux/2
  Demux/4 -> Mux/3
  Demux/1 -> Terminator/1
